simulink model "spring_mass_elem"  (R2013a)
settings: Solver=ode45  StartTime=0.0  StopTime=10.0  RelTol=1e-3
settings Model: Creator=d.alazard  LastModifiedBy=d.alazard

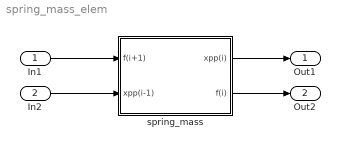
== system spring_mass_elem ==
  In1 : Inport
  In2 : Inport  Port=2
  spring_mass : Subsystem  mask{m=0.1, k=2}
      mask prompts: m "Mass"; k "Stiffness"
  Out1 : Outport
  Out2 : Outport  Port=2
  wires:
  In1/1 -> spring_mass/1(f(i+1))
  In2/1 -> spring_mass/2(xpp(i-1))
  spring_mass/1(xpp(i)) -> Out1/1
  spring_mass/2(f(i)) -> Out2/1

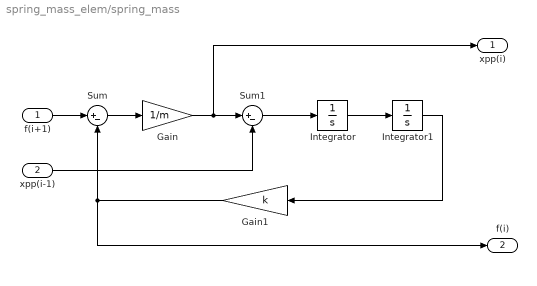
== system spring_mass_elem/spring_mass ==
  f(i+1) : Inport
  xpp(i-1) : Inport  Port=2
  Gain : Gain  Gain=1/m
  Gain1 : Gain  Gain=k
  Integrator : Integrator
  Integrator1 : Integrator
  Sum : Sum  Inputs=|+-
  Sum1 : Sum  Inputs=|+-
  xpp(i) : Outport
  f(i) : Outport  Port=2
  wires:
  xpp(i-1)/1 -> Sum1/2
  f(i+1)/1 -> Sum/1
  Integrator1/1 -> Gain1/1
  Sum1/1 -> Integrator/1
  Integrator/1 -> Integrator1/1
  Sum/1 -> Gain/1
  Gain/1 -> xpp(i)/1, Sum1/1
  Gain1/1 -> f(i)/1, Sum/2
